simulink model "navigation_filter"  (R2024b)
settings: Solver=FixedStepAuto  StartTime=0.0  StopTime=200.0  FixedStep=ST  RelTol=1e-3
values from neighbouring files (symbols this model uses):
  bias_gyro = [0.02 0.01 0.007]    [sensors.m]    (also in sensors_2.m = [0.2 0.1 0])
  dt = ST    (= 0.01)    [WP_gen.m]
  freq_acc = 50    [sensors.m]    (also in sensors_2.m)
  freq_gyro = 10    [sensors.m]    (also in sensors_2.m)
  freq_UWB = freq_gyro    (= 10)    [sensors.m]    (also in sensors_2.m)
  g = 9.81    [trajectory_gen_cartesian.m]
  N_bases = size(P_bases_ned, 1)    [sensors.m]    (also in sensors_2.m)
  pos_ned = [pos_ned_n pos_ned_e pos_ned_d]    [WP_gen.m]    (also in trajectory_gen_cartesian.m = pos_n_filt)
  Q = 100*diag([q_pos_1, q_pos_2, q_pos_3, q_vel_1, q_vel_2, q_vel_3, q_acc_1,q_acc_2,q_acc_3, q_quat_1, q_quat_2, q_quat_3, q_quat_4, q_omega_1, q_omega_2, q_omega_3, q_bias_1, q_bias_2, q_bias_3])    [sensors.m]    (also in sensors_2.m)
  Q_att = 100*diag([q_roll, q_pitch, q_yaw, q_omega_1, q_omega_2, q_omega_3, q_bias_1, q_bias_2, q_bias_3])    [sensors_2.m]
  quat_c_b = compact(quat_b)    [trajectory_gen_cartesian.m]
  sensor_covariances = [UWB_cov, ACC_cov, MAG_cov, GYRO_cov]    [sensors.m]    (also in sensors_2.m)
  ST = 1/100    (= 0.01)    [WP_gen.m]
  std_dev_accx = 0.02    [sensors.m]    (also in sensors_2.m = 0.01)
  std_dev_accy = 0.02    [sensors.m]    (also in sensors_2.m = 0.01)
  std_dev_accz = 0.02    [sensors.m]    (also in sensors_2.m = 0.01)
  std_dev_gyro1 = 1e-7    (= 1e-07)    [sensors.m]    (also in sensors_2.m = 3e-06)
  std_dev_gyro2 = 1e-7    (= 1e-07)    [sensors.m]    (also in sensors_2.m = 3e-06)
  std_dev_gyro3 = 1e-7    (= 1e-07)    [sensors.m]    (also in sensors_2.m = 3e-06)
  std_dev_magx = 0.03    [sensors.m]    (also in sensors_2.m)
  std_dev_magy = 0.03    [sensors.m]    (also in sensors_2.m)
  std_dev_magz = 0.03    [sensors.m]    (also in sensors_2.m)
  std_dev_UWB1 = 1e-6    (= 1e-06)    [sensors.m]    (also in sensors_2.m)
  Tf = ST    [sensors.m]    (also in sensors_2.m)
  vel_n = vel_n_filt    [trajectory_gen_cartesian.m]
undefined symbols (not defined in the file or in its folder): DiscIntNeverNeededParam
libraries: cstblocks x8, simulink x3, aerolibutil x2
(part 2 of 2)

== matlab function navigation_filter/Filter_attitute_euler ==
  data: mag_meas input; x_out output; omega_meas input; Q_att parameter; dt parameter; sensor_covariances parameter
function x_out = filter_attitude(mag_meas, omega_meas, Q_att, dt, sensor_covariances)
    %% definition of variables
    % state vector - [eul(3), omega(3), gyro_bias(3)] -> 9-dim

    persistent P % covariance matrix 
    persistent x 

    %% Initialization
    if isempty(P)   % this is done in the first cycle --> the persistent variables are initialized
        P = 10*Q_att;
        P(7:9,7:9) = P(7:9,7:9)*10^5; % apriori estimate of gyro bias is bad
        
        x = zeros(9,1);
        x(1:3) = [0; 0; 0]; % initial Euler angles: roll, pitch, yaw
        x(4:6) = omega_meas;
    end

    %% Prediction
    [x, P] = prediction(x, dt, Q_att, P);

    %% Correction
    [x, P] = correction(x, P, mag_meas, omega_meas, sensor_covariances);
    x_out = x;

end

function [x, P] = prediction(x, dt, Q_att, P)
    % state vector: [roll, pitch, yaw, omega(3), gyro_bias(3)]
    roll = x(1); pitch = x(2); yaw = x(3);
    w_x = x(4); w_y = x(5); w_z = x(6);
    byas_gx = x(7); byas_gy = x(8); byas_gz = x(9);

    % Remove bias from omega
    omega = [w_x; w_y; w_z];

    % Compute angular rate to Euler rate transformation (ZYX)
    T = [1 sin(roll)*tan(pitch) cos(roll)*tan(pitch);
         0 cos(roll)            -sin(roll);
         0 sin(roll)/cos(pitch) cos(roll)/cos(pitch)];

    eul_dot = T * omega;

    % Update Euler angles
    eul = [roll; pitch; yaw] + eul_dot * dt;

    % Wrap yaw to [-pi, pi]
    eul(1) = wrapToPi(eul(1));
    eul(2) = wrapToPi(eul(2));
    eul(3) = wrapToPi(eul(3));

    x = [eul; w_x; w_y; w_z; byas_gx; byas_gy; byas_gz];

    % Update covariance (simple prediction step for example)
    P = 10*Q_att;
end

function [x, P] = correction(x, P, mag_meas, omega_meas, sensor_covariances)
    % state vector: [roll, pitch, yaw, omega(3), gyro_bias(3)]
    roll = x(1); pitch = x(2); yaw = x(3);
    w_x = x(4); w_y = x(5); w_z = x(6);
    byas_gx = x(7); byas_gy = x(8); byas_gz = x(9);
    % sensor_covariances = [UWB(pos_n, pos_e, pos_d), Acc (acc_x, acc_y, acc_z), Mag (n, e, d), gyro (wx, wy, wz)]

    
    % gyro
    pred_gyro_x = w_x + byas_gx;
    pred_gyro_y = w_y + byas_gy;
    pred_gyro_z = w_z + byas_gz;

    %% y_meas & y_pred
    % mag
    mag_n = [0.24 0 0.40]'; % approx Gauss field, no declination 

    %compute Cnb
    Cz=[cos(yaw)     sin(yaw)     0; ...
        -sin(yaw)    cos(yaw)     0; ...
        0               0               1];
    Cy=[cos(pitch)     0               -sin(pitch); ...
        0               1               0; ...
        sin(pitch)     0               cos(pitch)];
    Cx=[1               0               0;...
        0               cos(roll)     sin(roll); ...
        0               -sin(roll)    cos(roll)];
    Cnb = (Cx*Cy*Cz);
    mag_b = Cnb*mag_n;

    y_meas = [mag_meas', omega_meas'];
    y_pred = [mag_b', pred_gyro_x, pred_gyro_y, pred_gyro_z];

    %% H
    H = H_matrix_only_attitude(x);

    %% Correction step
    covariances = sensor_covariances(7:12);
    R = diag(covariances);

    e = (y_meas - y_pred)';
    S = H*P*H' + R;
    L = P*H'*pinv(S);
    corr = L*e;
    x = x + corr;
    P = (eye(9) - L*H)*P*(eye(9) - L*H)' + L*R*L';


end

== matlab function navigation_filter/MATLAB Function4 ==
  data: q input size=4; euler output
function euler = quat2euler(q)
    euler = -quat2eul(q', "XYZ");
    % euler = rad2deg(euler);
end

% function euler = quat2euler(q)
% % quat2euler Convert quaternion to Euler angles (roll, pitch, yaw)
% % Input:  
% %   q - quaternion as a 1x4 vector [w x y z] or Nx4 matrix
% % Output: 
% %   euler - Nx3 matrix of Euler angles [roll pitch yaw] in radians
% 
%     if size(q, 1) ~= 4
%         error('Quaternion must be a Nx4 matrix: [w x y z]');
%     end
% 
%     % Normalize quaternion
%     q = q ./ vecnorm(q, 2, 2);
% 
%     w = q(1);
%     x = q(2);
%     y = q(3);
%     z = q(4);
% 
%     % Compute roll
%     roll = atan2(2*(w.*x + y.*z), 1 - 2*(x.^2 + y.^2));
% 
%     % Compute pitch (with clipping)
%     sinp = 2*(w.*y - z.*x);
%     sinp = max(min(sinp, 1), -1);  % clip to [-1, 1]
%     pitch = asin(sinp);
% 
%     % Compute yaw
%     yaw = atan2(2*(w.*z + x.*y), 1 - 2*(y.^2 + z.^2));
% 
%     euler = [roll, pitch, yaw];
% end

== matlab function navigation_filter/q2eul__ ==
  data: u input; y output
function y = fcn(u)
    y = quat2eul(u,"ZYX");
    y = rad2deg(y);

== matlab function navigation_filter/MATLAB Function6 ==
  data: q input; rpy output
function rpy = quat2rpy(q)
% quat2rpy - Converte un quaternione in [roll, pitch, yaw] in radianti
% INPUT:
%   q : quaternion object (singolo)
% OUTPUT:
%   rpy : 1x3 vector [roll, pitch, yaw] in radianti

    % Estrai i componenti del quaternione
    q0 = q(1);  % scalare
    q1 = q(2);
    q2 = q(3);
    q3 = q(4);

    % Calcolo angoli
    % roll (x-axis rotation)
    sinr_cosp = 2*(q0*q1 + q2*q3);
    cosr_cosp = 1 - 2*(q1^2 + q2^2);
    roll = atan2(sinr_cosp, cosr_cosp);

    % pitch (y-axis rotation)
    sinp = 2*(q0*q2 - q3*q1);
    if abs(sinp) >= 1
        pitch = sign(sinp)*pi/2;  % saturazione
    else
        pitch = asin(sinp);
    end

    % yaw (z-axis rotation)
    siny_cosp = 2*(q0*q3 + q1*q2);
    cosy_cosp = 1 - 2*(q2^2 + q3^2);
    yaw = atan2(siny_cosp, cosy_cosp);

    rpy = [roll, pitch, yaw];
end

== matlab function navigation_filter/UWB sensor 10Hz/Distances computation ==
  data: pos_ned input; d output; P_bases_ned parameter
function d = dist_comp(pos_ned, P_bases_ned)
% Calcola le distanze tra la posizione stimata e ciascuna base UWB
%
% Input:
%   pos_ned:       vettore 3x1 [x; y; z]
%   P_bases_ned:   matrice Nx3 con le posizioni delle basi (ogni riga è una base)
%
% Output:
%   d:             vettore Nx1 con le distanze calcolate

N = size(P_bases_ned, 1);  % numero di basi
d = zeros(N, 1);

for i = 1:N
    Pi = P_bases_ned(i, :)';
    d(i) = norm(pos_ned - Pi);
end

% function d = dist_comp(pos_ned, P_base1_ned, P_base2_ned, P_base3_ned, P_base4_ned)
% d = [ norm(pos_ned-P_base1_ned); 
%       norm(pos_ned-P_base2_ned);
%       norm(pos_ned-P_base3_ned);
%       norm(pos_ned-P_base4_ned) ];

== matlab function navigation_filter/Subsystem/make Cbn ==
  data: q input; R_nb output
function R_nb = quat2rotmat(q)
%QUAT2ROTMAT Converts a quaternion to rotation matrix from body to navigation frame
%   q: 1x4 vector [w x y z], representing orientation of body w.r.t. navigation frame
%   R_nb: 3x3 rotation matrix from body to navigation

% Normalize quaternion to be safe
q = q / norm(q);
w = q(1); x = q(2); y = q(3); z = q(4);

% Rotation matrix from body to navigation frame (passive rotation)
R_nb = [ ...
    1 - 2*(y^2 + z^2),     2*(x*y - z*w),       2*(x*z + y*w);
    2*(x*y + z*w),         1 - 2*(x^2 + z^2),   2*(y*z - x*w);
    2*(x*z - y*w),         2*(y*z + x*w),       1 - 2*(x^2 + y^2)];
end

== matlab function navigation_filter/Subsystem1/make Cbn ==
  data: q input; R_nb output
function R_nb = quat2rotmat(q)
%QUAT2ROTMAT Converts a quaternion to rotation matrix from body to navigation frame
%   q: 1x4 vector [w x y z], representing orientation of body w.r.t. navigation frame
%   R_nb: 3x3 rotation matrix from body to navigation

% Normalize quaternion to be safe
q = q / norm(q);
w = q(1); x = q(2); y = q(3); z = q(4);

% Rotation matrix from body to navigation frame (passive rotation)
R_nb = [ ...
    1 - 2*(y^2 + z^2),     2*(x*y - z*w),       2*(x*z + y*w);
    2*(x*y + z*w),         1 - 2*(x^2 + z^2),   2*(y*z - x*w);
    2*(x*z - y*w),         2*(y*z + x*w),       1 - 2*(x^2 + y^2)];
end

== matlab function navigation_filter/make Cnb ==
  data: Q_NB input; mag_b output
function mag_b = sim_mag_body(Q_NB)

%define magnetic field and rotate to bodyframe

mag_n = [0.24; 0; 0.40];            % [G], approx Gauss field
Rm_N2B = quaternion2matrix(Q_NB);
mag_b = Rm_N2B * mag_n;

== matlab function navigation_filter/Attitude Mechnization1/quaternion update ==
  data: omega_meas input; q_NB input; q_NB_p output; ST parameter
function q_NB_p = fcn(omega_meas, q_NB, ST)
% This function returns the quaternion of the rotation from Navigation to Body

delta_angle = omega_meas .* ST;       % angle variation in 1 step
delta_q = eul2quat([delta_angle(3), delta_angle(2), delta_angle(1)]);   % angle variation in quaternion form (rotation composition ZYX)

% Rotation composition as quaternion multiplication
q_NB_p = q_multi(q_NB, delta_q);

== matlab function navigation_filter/Attitude Mechnization3/quaternion update ==
  data: omega_meas input; q_NB input; q_NB_p output; ST parameter
function q_NB_p = fcn(omega_meas, q_NB, ST)

delta_angle = omega_meas .* ST;       % angle variation in 1 step
delta_q = eul2quat([delta_angle(3), delta_angle(2), delta_angle(1)]);   % angle variation in quaternion form (rotation composition ZYX)

% Rotation composition as quaternion multiplication
q_NB_p = q_multi(q_NB, delta_q);

== matlab function navigation_filter/Attitude Mechnization2/quaternion update ==
  data: omega_meas input; q_NB input; q_NB_p output; ST parameter
function q_NB_p = fcn(omega_meas, q_NB, ST)

delta_angle = omega_meas .* ST;       % angle variation in 1 step
delta_q = eul2quat([delta_angle(3), delta_angle(2), delta_angle(1)]);   % angle variation in quaternion form (rotation composition ZYX)

% Rotation composition as quaternion multiplication
q_NB_p = q_multi(q_NB, delta_q);

== matlab function navigation_filter/MATLAB Function ==
  data: q input size=4; euler output
function euler = quat2euler(q)
    euler = -quat2eul(q', "XYZ");
    % euler = rad2deg(euler);
end

% function euler = quat2euler(q)
% % quat2euler Convert quaternion to Euler angles (roll, pitch, yaw)
% % Input:  
% %   q - quaternion as a 1x4 vector [w x y z] or Nx4 matrix
% % Output: 
% %   euler - Nx3 matrix of Euler angles [roll pitch yaw] in radians
% 
%     if size(q, 1) ~= 4
%         error('Quaternion must be a Nx4 matrix: [w x y z]');
%     end
% 
%     % Normalize quaternion
%     q = q ./ vecnorm(q, 2, 2);
% 
%     w = q(1);
%     x = q(2);
%     y = q(3);
%     z = q(4);
% 
%     % Compute roll
%     roll = atan2(2*(w.*x + y.*z), 1 - 2*(x.^2 + y.^2));
% 
%     % Compute pitch (with clipping)
%     sinp = 2*(w.*y - z.*x);
%     sinp = max(min(sinp, 1), -1);  % clip to [-1, 1]
%     pitch = asin(sinp);
% 
%     % Compute yaw
%     yaw = atan2(2*(w.*z + x.*y), 1 - 2*(y.^2 + z.^2));
% 
%     euler = [roll, pitch, yaw];
% end

== matlab function navigation_filter/UWB sensor 10Hz/UWB position computation ==
  data: d_meas input; UWB_pos_ned output size=3; P_bases_ned parameter
function UWB_pos_ned = pos_comp_6bases(d_meas, P_bases_ned)
% Calcola la posizione UWB in coordinate NED utilizzando 6 basi,
% usando la prima base come riferimento.
%
% Input:
%   d_meas:        vettore 6x1 con le distanze misurate [d1; d2; ...; d6]
%   P_bases_ned:   matrice 6x3, ogni riga è una base [x y z]
%
% Output:
%   UWB_pos_ned:   posizione stimata [x; y; z]

% Riferimento: base 1
Pref = P_bases_ned(1, :)';
dref = d_meas(1);

% Costruzione delle matrici A e C usando le altre 5 basi
A = zeros(5, 3);
C = zeros(5, 1);

for i = 2:6
    Pi = P_bases_ned(i, :)';
    di = d_meas(i);
    
    A(i-1, :) = (Pi - Pref)';
    C(i-1) = dref^2 - di^2 - sum(Pref.^2) + sum(Pi.^2);
end

% Soluzione ai minimi quadrati
UWB_pos_ned = 0.5 * pinv(A) * C;  % oppure: 0.5 * A \ C

% function UWB_pos_ned = pos_comp(d_meas, P_base1_ned, P_base2_ned, P_base3_ned, P_base4_ned)
% 
% % Formula to compute the position knowing the distances: X = 1/2 * inv(A' * A) * A' * C
% % (from "Research on UWB indoor 3D positioning algorithm based on the least squares method")
% 
% d1 = d_meas(1);
% d2 = d_meas(2);
% d3 = d_meas(3);
% d4 = d_meas(4);
% 
% A = [(P_base1_ned-P_base4_ned)';
%      (P_base2_ned-P_base4_ned)';
%      (P_base3_ned-P_base4_ned)' ];
% 
% C = [d4^2-d1^2-sum(P_base4_ned.^2)+sum(P_base1_ned.^2);
%      d4^2-d2^2-sum(P_base4_ned.^2)+sum(P_base2_ned.^2);
%      d4^2-d3^2-sum(P_base4_ned.^2)+sum(P_base3_ned.^2)];
% 
% % UWB_pos_ned = 1/2 * inv(A' * A) * A' * C;
% UWB_pos_ned = 1/2 * pinv(A) * C;

== matlab function navigation_filter/Navigation Filter ==
  data: flag10Hz input; flag50Hz input; flagINITOK input; bias_gyro_removed input; xout output; measure input; Pout output; sensor_covariances parameter; Q parameter; dt parameter; quat_c_b parameter; g parameter
function [xout,Pout] = navigation_KF(flag10Hz, flag50Hz, flagINITOK, bias_gyro_removed, measure, sensor_covariances, Q, dt, quat_c_b, g)
% state vector - [pos(3), vel(3), acc(3), q(4), omega(3), gyro_bias(3)] -> 19-dim
% Measure = 13-dimensional vector
% measure = [UWB(pos_n, pos_e, pos_d), Acc (acc_x, acc_y, acc_z), Mag (n, e, d), gyro (wx, wy, wz)]

%% definition of variables
persistent P % covariance matrix 
persistent x 
persistent filter_running
if isempty(P)   % this is done in the first cycle --> the persistent variables are inititialized
    P = single(0.1)*Q;
    P(4:6,4:6) = P(4:6,4:6)*10; % apriori esteem of velocity are bad
    P(17:19,17:19) = P(17:19,17:19)*1e3; % apriori esteem of biases are bad
    P(19,19) = P(19,19)*1e-2;

    x = single(zeros(19,1));
    x(10) = 1; % element of the quaternion q_w = 1

    filter_running = logical(false); % filter starts in OFF, must wait for flagINITOK to become true
end

%% initialization 
if ~filter_running && flagINITOK      
    % if filter is not running and initialization can be performed -> this
    % "if" is computed only one time, as soon as the bias of the gyro is
    % obtained
    
    % initialize state
    % x(1:3) = measure(1:3);  % pos from UWB
    % x(4:6) = [0, 0, 0];     % velocity is not known
    % x(7:9) = measure(4:6);  % acc from ACC
    % x(10:13) = [1,0,0,0]; %[quat_c(1,1), quat_c(1,2), quat_c(1,3), quat_c(1,4)];%[1,0,0,0];   % initial quaternion
    % x(14:16) = measure(10:12) - bias_gyro_removed ; % omega from gyroscope
    % x(17:19) = bias_gyro_removed;
    x(19) = bias_gyro_removed(3);


    % x(4) = measure(end);

    % set filter as running
    filter_running = true;
end


if filter_running
    %% select update type
    if(flag10Hz && flag50Hz) % all sensors
        fuse = 1;
        disp("fuse = 1")
    elseif(flag10Hz) % Gyro & UWB
        fuse = 2;
        disp("fuse = 2")
    elseif(flag50Hz) % Acc & Mag
        fuse = 3;
        disp("fuse = 3")
    else % nothing - only prediction
        fuse = 4;
    end

    %% Prediction
    [x, P] = prediction(x, dt, Q, P, g);

    %% Correction
    [x, P] = correction(x, P, measure, sensor_covariances, fuse, g);

end

xout = x;
Pout = P;
end

% ----------------------------------------------------------------------------------

function [x, P] = prediction(x, dt, Q, P, g)
% update the predicted state
    north = x(1); east = x(2); down = x(3);         % pos (NED)
    vel_n = x(4); vel_e = x(5); vel_d = x(6);       % vel (nav frame)
    acc_x = x(7); acc_y = x(8); acc_z = x(9);       % acc (body frame)
    qw = x(10); qx = x(11); qy = x(12); qz = x(13); % quaternion (from nav to body)
    w_x = x(14); w_y = x(15); w_z = x(16);          % omega (body)
    byas_gx = x(17); byas_gy = x(18); byas_gz = x(19);% byass gyro

    % convert acc from body to navigation frame
    R_nb = quaternion2matrix([qw, qx, qy, qz]);     % rotation from body to nav
    acc_ned = R_nb * [acc_x; acc_y; acc_z];
    acc_n = acc_ned(1);
    acc_e = acc_ned(2);
    acc_d = acc_ned(3);
    
    % acc
    % acc_d = acc_d - g; % gravity compensation

    % positions
    north = north + vel_n*dt + 0.5*acc_n*dt^2;
    east = east + vel_e*dt + 0.5*acc_e*dt^2 ;
    down = down + vel_d*dt + 0.5*acc_d*dt^2;

    % vel
    vel_n = vel_n + acc_n*dt;
    vel_e = vel_e + acc_e*dt;
    vel_d = vel_d + acc_d*dt;

    % attitude - quaternion update
    d_ang = [w_x; w_y; w_z] .* dt;  % delta angle (euler) 
    d_q = eul2quat([d_ang(3), d_ang(2), d_ang(1)]);  % delta angle (quaternion)
    new_quat = q_multi([qw,qx,qy,qz],d_q);
    q_w = new_quat(1);
    q_x = new_quat(2);
    q_y = new_quat(3);
    q_z = new_quat(4);

    % output:
    x = [north, east, down, vel_n, vel_e, vel_d, acc_x, acc_y, acc_z, new_quat, w_x, w_y, w_z, byas_gx, byas_gy, byas_gz]';

    % P
    F = single(F_matrix(north,east,down,vel_n,vel_e,vel_d,acc_x,acc_y,acc_z,q_w,q_x,q_y,q_z,w_x,w_y,w_z,byas_gx,byas_gy,byas_gz,dt));
    P = F*P*F' + Q;
    
end
  
function [x, P] = correction(x, P, measure, covariances, fuse,g)
    H_tot = single(H_matrix(x));
    y_pred_tot = get_y_pred(x,g);
    

    % Measure = 12-dimensional vector
    % measure = [UWB(pos_n, pos_e, pos_d), Acc (acc_x, acc_y, acc_z), Mag (n, e, d), gyro (wx, wy, wz)]

    switch fuse
        case 1             
            % all measurements, including pitot
            % y = measure;
            % y_pred = y_pred_tot;
            % H = H_tot;
            % R = diag( horzcat(covariances, covariances(1)) );
            % 
            % e = y - y_pred;
            % S = H*P*H' + R;
            % L = P*H'*pinv(S);
            % corr = L*e;
            % x = x + corr;
            % P = (eye(19) - L*H)*P*(eye(19) - L*H)' + L*R*L';
            
            % All measures except pitot
            y = measure(1:12);
            y_pred = y_pred_tot(1:12);
            H = H_tot(1:12,:);
            R = diag(covariances);
            R(10:12,10:12) = R(10:12,10:12) * 5;

            e = y - y_pred;
            S = H*P*H' + R;
            L = P*H'*pinv(S);
            corr = L*e;
            x = x + corr;
            P = (eye(19) - L*H)*P*(eye(19) - L*H)' + L*R*L';
        case 2
            % Measurements of UWB & Gyro
            y = [measure(1:3); measure(10:12)];
            y_pred = [ y_pred_tot(1:3); y_pred_tot(10:12) ];
            H = [H_tot(1:3,:); H_tot(10:12,:)];
            R = diag([covariances(1:3), covariances(10:12)*5]);

            e = y - y_pred;
            S = H*P*H' + R;
            L = P*H'*pinv(S);
            corr = L*e;
            x = x + corr;
            P = (eye(19) - L*H)*P*(eye(19) - L*H)' + L*R*L';
        case 3
            % Measurements of Acc & Mag
            y = [measure(4:9)];
            y_pred = y_pred_tot(4:9);
            H = [H_tot(4:9, :)];
            R = diag([covariances(4:9)]);

            e = y - y_pred;
            S = H*P*H' + R;
            L = P*H'*pinv(S);
            corr = L*e;
            x = x + corr;
            P = (eye(19) - L*H)*P*(eye(19) - L*H)' + L*R*L';
    end

end
